simulink model "filter_acc"  (R2023b)
settings: Solver=VariableStepAuto  StartTime=0.0  StopTime=10.0  RelTol=1e-3
values from neighbouring files (symbols this model uses):
  Ts_slk = 0.01    [main_matteo.m]    (also in quadcopterMain.m)
undefined symbols (not defined in the file or in its folder): meas_pole
settings Model: Creator=teoma  LastModifiedBy=teoma

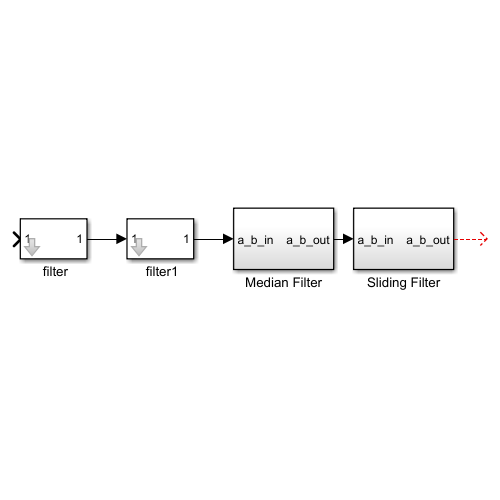
[thumbnail: Simulink's stored preview of the top-level diagram]
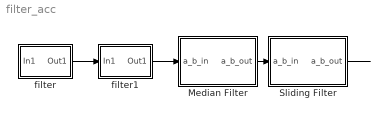
== system filter_acc ==
  " filter" : Subsystem  mask{p=5}
      mask prompts: p "pole (p)"
  " filter1" : Subsystem  mask{p=meas_pole}
      mask prompts: p "pole (p)"
  Median Filter : Subsystem
  Sliding Filter : Subsystem
  wires:
  Sliding Filter/1(a_b_out) -> ?
  Median Filter/1(a_b_out) -> Sliding Filter/1(a_b_in)
  " filter"/1(Out1) -> " filter1"/1(In1)
  " filter1"/1(Out1) -> Median Filter/1(a_b_in)

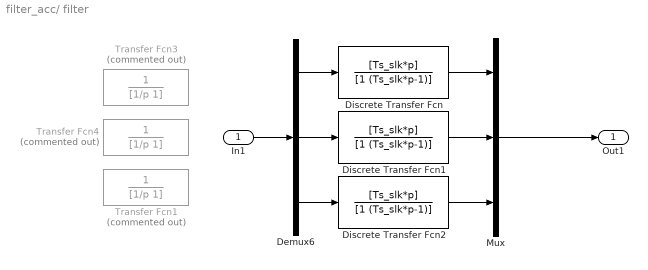
== system filter_acc/ filter ==
  In1 : Inport
  Demux6 : Demux  Outputs=3
  Discrete Transfer Fcn : DiscreteTransferFcn  Numerator=[Ts_slk*p]  Denominator=[1 (Ts_slk*p-1)]
  Discrete Transfer Fcn1 : DiscreteTransferFcn  Numerator=[Ts_slk*p]  Denominator=[1 (Ts_slk*p-1)]
  Discrete Transfer Fcn2 : DiscreteTransferFcn  Numerator=[Ts_slk*p]  Denominator=[1 (Ts_slk*p-1)]
  Mux : Mux  Inputs=3
  Transfer Fcn1 : TransferFcn  Commented=on  Denominator=[1/p 1]
  Transfer Fcn3 : TransferFcn  Commented=on  Denominator=[1/p 1]
  Transfer Fcn4 : TransferFcn  Commented=on  Denominator=[1/p 1]
  Out1 : Outport
  wires:
  Discrete Transfer Fcn1/1 -> Mux/2
  Demux6/3 -> Discrete Transfer Fcn2/1
  Mux/1 -> Out1/1
  Discrete Transfer Fcn2/1 -> Mux/3
  Discrete Transfer Fcn/1 -> Mux/1
  In1/1 -> Demux6/1
  Demux6/1 -> Discrete Transfer Fcn/1
  Demux6/2 -> Discrete Transfer Fcn1/1

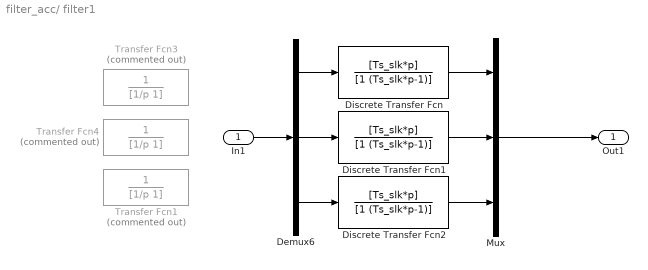
== system filter_acc/ filter1 ==
  In1 : Inport
  Demux6 : Demux  Outputs=3
  Discrete Transfer Fcn : DiscreteTransferFcn  Numerator=[Ts_slk*p]  Denominator=[1 (Ts_slk*p-1)]
  Discrete Transfer Fcn1 : DiscreteTransferFcn  Numerator=[Ts_slk*p]  Denominator=[1 (Ts_slk*p-1)]
  Discrete Transfer Fcn2 : DiscreteTransferFcn  Numerator=[Ts_slk*p]  Denominator=[1 (Ts_slk*p-1)]
  Mux : Mux  Inputs=3
  Transfer Fcn1 : TransferFcn  Commented=on  Denominator=[1/p 1]
  Transfer Fcn3 : TransferFcn  Commented=on  Denominator=[1/p 1]
  Transfer Fcn4 : TransferFcn  Commented=on  Denominator=[1/p 1]
  Out1 : Outport
  wires:
  Discrete Transfer Fcn1/1 -> Mux/2
  Demux6/3 -> Discrete Transfer Fcn2/1
  Mux/1 -> Out1/1
  Discrete Transfer Fcn2/1 -> Mux/3
  Discrete Transfer Fcn/1 -> Mux/1
  In1/1 -> Demux6/1
  Demux6/1 -> Discrete Transfer Fcn/1
  Demux6/2 -> Discrete Transfer Fcn1/1

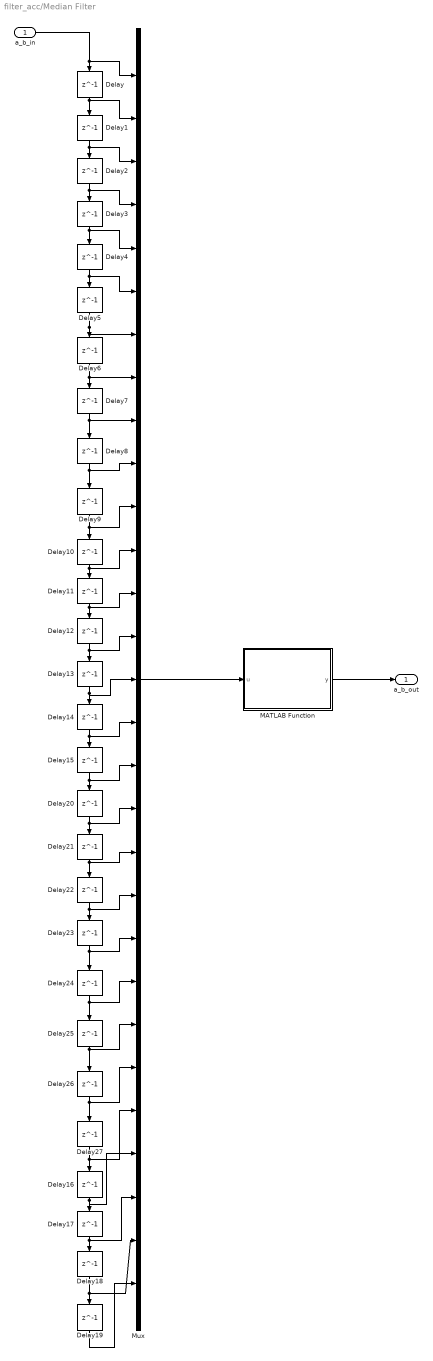
== system filter_acc/Median Filter ==
  a_b_in : Inport
  Delay{,1..27} (28 alike) : Delay  DelayLength=1  InitialCondition=zeros(1,3)  SampleTime=Ts_slk
  MATLAB Function : MATLAB Function  TreatAsAtomicUnit=on
  Mux : Mux  Inputs=29
  a_b_out : Outport
  wires:
  a_b_in/1 -> Delay/1, Mux/1
  Delay1/1 -> Delay2/1, Mux/3
  Delay2/1 -> Delay3/1, Mux/4
  Delay/1 -> Delay1/1, Mux/2
  Delay3/1 -> Delay4/1, Mux/5
  Mux/1 -> MATLAB Function/1(u)
  MATLAB Function/1(y) -> a_b_out/1
  Delay4/1 -> Delay5/1, Mux/6
  Delay5/1 -> Delay6/1, Mux/7
  Delay6/1 -> Delay7/1, Mux/8
  Delay8/1 -> Mux/10, Delay9/1
  Delay11/1 -> Mux/13, Delay12/1
  Delay12/1 -> Mux/14, Delay13/1
  Delay7/1 -> Mux/9, Delay8/1
  Delay9/1 -> Delay10/1, Mux/11
  Delay10/1 -> Mux/12, Delay11/1
  Delay13/1 -> Mux/15, Delay14/1
  Delay24/1 -> Mux/22, Delay25/1
  Delay23/1 -> Mux/21, Delay24/1
  Delay20/1 -> Mux/18, Delay21/1
  Delay15/1 -> Mux/17, Delay20/1
  Delay21/1 -> Mux/19, Delay22/1
  Delay27/1 -> Mux/25, Delay16/1
  Delay18/1 -> Delay19/1, Mux/28
  Delay25/1 -> Mux/23, Delay26/1
  Delay22/1 -> Mux/20, Delay23/1
  Delay26/1 -> Mux/24, Delay27/1
  Delay14/1 -> Mux/16, Delay15/1
  Delay17/1 -> Mux/27, Delay18/1
  Delay16/1 -> Mux/26, Delay17/1
  Delay19/1 -> Mux/29

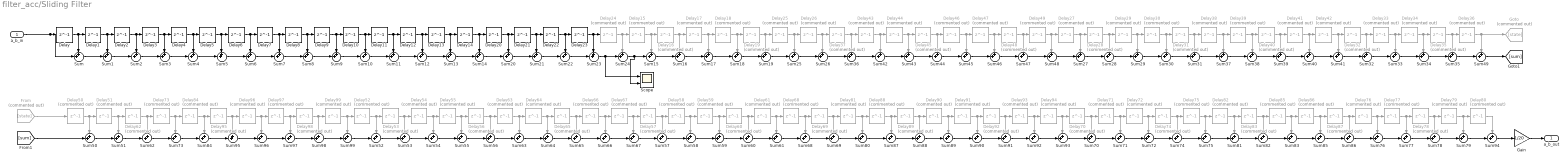
== system filter_acc/Sliding Filter ==
  a_b_in : Inport
  Delay{,1..14,20..23} (19 alike) : Delay  DelayLength=1  SampleTime=Ts_slk
  Delay{15..19,24..99} (81 alike) : Delay  Commented=on  DelayLength=1  SampleTime=Ts_slk
  From : From  Commented=on  GotoTag=state
  Gain : Gain  Gain=1/20
  Goto : Goto  Commented=on  GotoTag=state
  Scope : Scope  NumInputPorts=2
  Sum{,1..99} (100 alike) : Sum  Inputs=++|
  a_b_out : Outport
  wires:
  Delay/1 -> Sum/1, Delay1/1
  Delay1/1 -> Sum1/1, Delay2/1
  Delay2/1 -> Sum2/1, Delay3/1
  Delay3/1 -> Sum3/1, Delay4/1
  Sum/1 -> Sum1/2
  Sum1/1 -> Sum2/2
  Sum2/1 -> Sum3/2
  Sum3/1 -> Sum4/2
  Delay4/1 -> Delay5/1, Sum4/1
  Sum4/1 -> Sum5/2
  a_b_in/1 -> Sum/2, Delay/1
  Delay5/1 -> Sum5/1, Delay6/1
  Delay6/1 -> Sum6/1, Delay7/1
  Sum5/1 -> Sum6/2
  Sum6/1 -> Sum7/2
  Sum7/1 -> Sum8/2
  Delay7/1 -> Sum7/1, Delay8/1
  Delay8/1 -> Delay9/1, Sum8/1
  Delay9/1 -> Sum9/1, Delay10/1
  Delay10/1 -> Sum10/1, Delay11/1
  Delay11/1 -> Sum11/1, Delay12/1
  Delay12/1 -> Sum12/1, Delay13/1
  Delay13/1 -> Sum13/1, Delay14/1
  Sum11/1 -> Sum12/2
  Sum12/1 -> Sum13/2
  Sum13/1 -> Sum14/2
  Sum8/1 -> Sum9/2
  Sum9/1 -> Sum10/2
  Sum10/1 -> Sum11/2
  Delay14/1 -> Delay20/1, Sum14/1
  Delay19/1 -> Delay25/1, Sum19/1
  Sum16/1 -> Sum17/2
  Delay15/1 -> Sum15/1, Delay16/1
  Sum24/1 -> Scope/2, Sum15/2
  Sum17/1 -> Sum18/2
  Delay23/1 -> Delay24/1, Sum23/1
  Delay24/1 -> Sum24/1, Delay15/1
  Sum20/1 -> Sum21/2
  Delay22/1 -> Sum22/1, Delay23/1
  Delay18/1 -> Sum18/1, Delay19/1
  Sum23/1 -> Scope/1, Sum24/2
  Sum22/1 -> Sum23/2
  Sum14/1 -> Sum20/2
  Delay20/1 -> Sum20/1, Delay21/1
  Delay17/1 -> Sum17/1, Delay18/1
  Sum18/1 -> Sum19/2
  Delay21/1 -> Sum21/1, Delay22/1
  Delay16/1 -> Sum16/1, Delay17/1
  Sum15/1 -> Sum16/2
  Sum21/1 -> Sum22/2
  Sum41/1 -> Sum32/2
  Delay32/1 -> Sum32/1, Delay33/1
  Sum33/1 -> Sum34/2
  Delay42/1 -> Sum41/1, Delay32/1
  Sum37/1 -> Sum38/2
  Delay41/1 -> Delay42/1, Sum40/1
  Delay31/1 -> Delay38/1, Sum31/1
  Sum28/1 -> Sum29/2
  Delay28/1 -> Sum28/1, Delay29/1
  Delay27/1 -> Sum27/1, Delay28/1
  Delay49/1 -> Sum48/1, Delay27/1
  Sum48/1 -> Sum27/2
  Sum29/1 -> Sum30/2
  Delay48/1 -> Delay49/1, Sum47/1
  Sum44/1 -> Sum45/2
  Delay47/1 -> Sum46/1, Delay48/1
  Delay45/1 -> Sum44/1, Delay46/1
  Delay39/1 -> Sum38/1, Delay40/1
  Sum47/1 -> Sum48/2
  Delay38/1 -> Sum37/1, Delay39/1
  Sum40/1 -> Sum41/2
  Sum46/1 -> Sum47/2
  Sum34/1 -> Sum35/2
  Delay29/1 -> Sum29/1, Delay30/1
  Sum32/1 -> Sum33/2
  Delay40/1 -> Sum39/1, Delay41/1
  Delay46/1 -> Sum45/1, Delay47/1
  Delay33/1 -> Sum33/1, Delay34/1
  Sum27/1 -> Sum28/2
  Delay30/1 -> Sum30/1, Delay31/1
  Sum36/1 -> Sum42/2
  Delay44/1 -> Delay45/1, Sum43/1
  Sum39/1 -> Sum40/2
  Delay37/1 -> Sum36/1, Delay43/1
  Sum26/1 -> Sum36/2
  Sum43/1 -> Sum44/2
  Sum25/1 -> Sum26/2
  Delay35/1 -> Sum35/1, Delay36/1
  Sum42/1 -> Sum43/2
  Delay43/1 -> Sum42/1, Delay44/1
  Sum30/1 -> Sum31/2
  Sum45/1 -> Sum46/2
  Sum31/1 -> Sum37/2
  Delay26/1 -> Sum26/1, Delay37/1
  Delay25/1 -> Sum25/1, Delay26/1
  Delay34/1 -> Sum34/1, Delay35/1
  Sum38/1 -> Sum39/2
  Sum35/1 -> Sum49/2
  Sum19/1 -> Sum25/2
  Delay36/1 -> Goto/1, Sum49/1
  Sum49/1 -> [sum]
  Delay68/1 -> Sum68/1, Delay69/1
  Sum82/1 -> Sum83/2
  Sum68/1 -> Sum69/2
  Sum75/1 -> Sum81/2
  Delay88/1 -> Sum87/1, Delay89/1
  Delay79/1 -> Sum79/1, Delay80/1
  Sum74/1 -> Sum75/2
  Delay69/1 -> Sum69/1, Delay81/1
  Sum90/1 -> Sum91/2
  Sum83/1 -> Sum85/2
  Sum80/1 -> Sum87/2
  Sum88/1 -> Sum89/2
  Sum69/1 -> Sum80/2
  Sum70/1 -> Sum71/2
  Delay78/1 -> Sum78/1, Delay79/1
  Sum92/1 -> Sum93/2
  Sum78/1 -> Sum79/2
  Sum91/1 -> Sum92/2
  Sum85/1 -> Sum86/2
  Sum76/1 -> Sum77/2
  Delay72/1 -> Sum72/1, Delay74/1
  Delay82/1 -> Sum81/1, Delay83/1
  Sum72/1 -> Sum74/2
  Delay94/1 -> Sum93/1, Delay70/1
  Delay85/1 -> Sum83/1, Delay86/1
  Delay74/1 -> Sum74/1, Delay75/1
  Sum93/1 -> Sum70/2
  Delay90/1 -> Sum89/1, Delay91/1
  Delay92/1 -> Sum91/1, Delay93/1
  Delay93/1 -> Delay94/1, Sum92/1
  Delay75/1 -> Delay82/1, Sum75/1
  Sum71/1 -> Sum72/2
  Delay71/1 -> Sum71/1, Delay72/1
  Delay70/1 -> Sum70/1, Delay71/1
  Sum67/1 -> Sum57/2
  Delay57/1 -> Sum57/1, Delay58/1
  Sum58/1 -> Sum59/2
  Sum89/1 -> Sum90/2
  Delay61/1 -> Delay68/1, Sum61/1
  Delay67/1 -> Sum67/1, Delay57/1
  Sum63/1 -> Sum64/2
  Delay66/1 -> Delay67/1, Sum66/1
  Sum94/1 -> Gain/1
  Sum81/1 -> Sum82/2
  Sum77/1 -> Sum78/2
  Delay87/1 -> Sum86/1, Delay76/1
  Delay76/1 -> Sum76/1, Delay77/1
  Delay86/1 -> Delay87/1, Sum85/1
  Sum86/1 -> Sum76/2
  Sum53/1 -> Sum54/2
  Delay53/1 -> Sum53/1, Delay54/1
  Delay56/1 -> Delay63/1, Sum56/1
  Delay52/1 -> Sum52/1, Delay53/1
  Delay99/1 -> Sum99/1, Delay52/1
  Sum99/1 -> Sum52/2
  Sum54/1 -> Sum55/2
  Delay98/1 -> Delay99/1, Sum98/1
  Sum95/1 -> Sum96/2
  Delay97/1 -> Sum97/1, Delay98/1
  Delay95/1 -> Sum95/1, Delay96/1
  Delay55/1 -> Sum55/1, Delay56/1
  Sum98/1 -> Sum99/2
  Sum64/1 -> Sum65/2
  Delay64/1 -> Sum64/1, Delay65/1
  Delay58/1 -> Sum58/1, Delay59/1
  Delay81/1 -> Sum80/1, Delay88/1
  Delay63/1 -> Sum63/1, Delay64/1
  Sum66/1 -> Sum67/2
  Sum97/1 -> Sum98/2
  Delay77/1 -> Sum77/1, Delay78/1
  Sum59/1 -> Sum60/2
  Delay54/1 -> Sum54/1, Delay55/1
  Sum57/1 -> Sum58/2
  Delay89/1 -> Delay90/1, Sum88/1
  Delay65/1 -> Sum65/1, Delay66/1
  Delay96/1 -> Sum96/1, Delay97/1
  Sum52/1 -> Sum53/2
  From/1 -> Delay50/1
  Delay83/1 -> Sum82/1, Delay85/1
  Sum62/1 -> Sum73/2
  Delay84/1 -> Delay95/1, Sum84/1
  Sum65/1 -> Sum66/2
  Sum87/1 -> Sum88/2
  Delay62/1 -> Sum62/1, Delay73/1
  Sum51/1 -> Sum62/2
  Delay91/1 -> Sum90/1, Delay92/1
  Sum84/1 -> Sum95/2
  Sum50/1 -> Sum51/2
  Delay60/1 -> Sum60/1, Delay61/1
  Sum73/1 -> Sum84/2
  Delay73/1 -> Sum73/1, Delay84/1
  Sum55/1 -> Sum56/2
  Sum61/1 -> Sum68/2
  Delay80/1 -> Sum94/1
  Sum96/1 -> Sum97/2
  Sum79/1 -> Sum94/2
  Sum56/1 -> Sum63/2
  Delay51/1 -> Sum51/1, Delay62/1
  Delay50/1 -> Sum50/1, Delay51/1
  Delay59/1 -> Sum59/1, Delay60/1
  Sum60/1 -> Sum61/2
  Gain/1 -> a_b_out/1
  [sum] -> Sum50/2

== matlab function filter_acc/Median Filter/MATLAB Function ==
  data: u input; y output
function y = fcn(u)
[n,~] = size(u);
n = n/3;
norm = zeros(n,2);
for i = 1:1:n
    u_vect      = u(i*3-2:i*3,1); 
    norm(i,1)   = sqrt(u_vect'*u_vect);     % norm
    norm(i,2)   = i;                        % index
end
for i = 1:n-1
    for j = 1:n-i
        if norm(j,1) > norm(j+1,1)
            % Swap elements
            temp = norm(j,:);
            norm(j,:) = norm(j+1,:);
            norm(j+1,:) = temp;
        end
    end
end
indexMedian = floor(n/2-1);
median = norm(indexMedian,2);
y = u(median*3-2:median*3);
end
